simulink model "task5"  (R2023a)
settings: Solver=VariableStepAuto  StartTime=0.0  StopTime=10.0  RelTol=1e-3
settings Model: Creator=LENOVO  LastModifiedBy=LENOVO

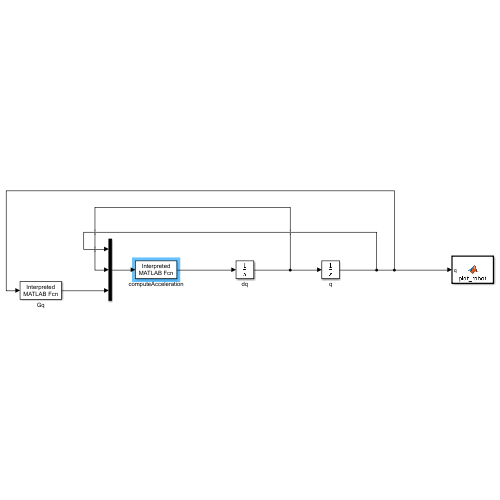
[thumbnail: Simulink's stored preview of the top-level diagram]
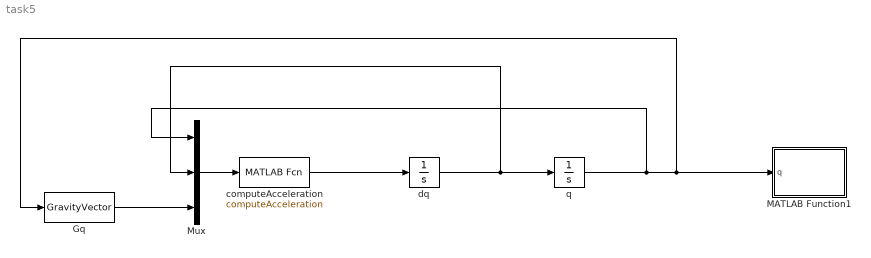
== system task5 ==
  Gq : MATLABFcn  MATLABFcn=GravityVector  OutputDimensions=2  Output1D=off
  MATLAB Function1 : MATLAB Function  TreatAsAtomicUnit=on
  Mux : Mux  Inputs=3
  computeAcceleration : MATLABFcn  MATLABFcn=computeAcceleration  OutputDimensions=2  Output1D=off
  dq : Integrator  InitialCondition=[0; 0]
  q : Integrator  InitialCondition=[pi/2; pi/4]
  wires:
  q/1 -> Mux/1, Gq/1, MATLAB Function1/1(q)
  Mux/1 -> computeAcceleration/1
  Gq/1 -> Mux/3
  dq/1 -> Mux/2, q/1
  computeAcceleration/1 -> dq/1

== matlab function task5/MATLAB Function1 ==
  data: q input
function plot_robot(q)
    % Link lengths
    q1 = q(1);
    q2 = q(2);
    l1 = 0.3; l2 = 0.2;
    
    % Joint positions
    x1 = l1 * cos(q1);
    y1 = l1 * sin(q1);
    x2 = x1 + l2 * cos(q1 + q2);
    y2 = y1 + l2 * sin(q1 + q2);
    
    % Plot
    plot([0, x1, x2], [0, y1, y2], '-o', 'LineWidth', 2);
    xlim([-0.6, 0.6]);
    ylim([-0.6, 0.6]);
    grid on;
    drawnow;
end
